simulink model "doc_filtercutoffs"  (R2014a)
settings: Solver=ode45  StartTime=0.0  StopTime=10.0  RelTol=1e-3
undefined symbols (not defined in the file or in its folder): commblksprivate, Info
libraries: commanapbnd3 x2
settings Model: ExtModeAutoUpdateStatusClock=off  Creator=The MathWorks Inc.
settings DataIOCC: SignalLoggingSaveFormat=ModelDataLogs  SignalLoggingName=logsOut
settings OptimizationCC: BlockReduction=off  BooleanDataType=off  ExpressionDepthLimit=2147483647  InitFltsAndDblsToZero=on
settings DebuggingCC: SaveWithParameterizedLinksMsg=none  UnderspecifiedInitializationDetection=Classic  SignalResolutionControl=TryResolveAllWithWarning  SolverPrmCheckMsg=none  MultiTaskDSMMsg=warning  MultiTaskCondExecSysMsg=none  FcnCallInpInsideContextMsg=UseLocalSettings  StateNameClashWarn=warning  StrictBusMsg=None
settings HardwareCC: ProdHWDeviceType=Specified
settings RTWCC: IncludeERTFirstTime=on
settings CodeAppCC: MangleLength=5
settings GRTTargetCC: TargetFcnLib=ansi_tfl_tmw.mat  CombineOutputUpdateFcns=off  GRTInterface=on

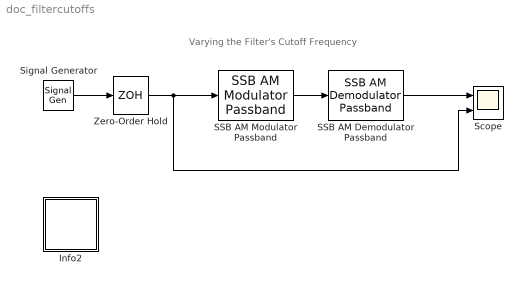
== system doc_filtercutoffs ==
  note: Varying the Filter's Cutoff Frequency
  Info2 : Subsystem  AncestorBlock=commblksprivate/Info  mask(Info){}
      settings: OpenFcn=helpview([docroot '/toolbox/comm/comm.map'], 'doc_filtercutoffs')
      mask Display: disp('Info')
  SSB AM Demodulator Passband : commanapbnd3/SSB AM Demodulator Passband  Fc=25  Ph=0  method=Butterworth  n=2  cf=30  Rp=0.1  Rs=50
  SSB AM Modulator Passband : commanapbnd3/SSB AM Modulator Passband  Fc=25  Ph=0  Sd=Upper  Ho=200
  Scope : Scope  NumInputPorts=2
      settings: YMin=-5~-5  YMax=5~5
  Signal Generator : SignalGenerator  WaveForm=sawtooth  Amplitude=4  Frequency=.3
  Zero-Order Hold : ZeroOrderHold  SampleTime=.01
  wires:
  Signal Generator/1 -> Zero-Order Hold/1
  SSB AM Modulator Passband/1 -> SSB AM Demodulator Passband/1
  SSB AM Demodulator Passband/1 -> Scope/1
  Zero-Order Hold/1 -> SSB AM Modulator Passband/1, Scope/2

== system doc_filtercutoffs/Info2 ==
